simulink model "im_model_exercise_version"  (Simulink 9.2)
settings: Solver=ode45  StartTime=0.0  StopTime=2  MaxStep=300e-6  RelTol=1e-5  EnableMultiTasking=on
InitFcn:
  | Motor_parameters_project
values from neighbouring files (symbols this model uses):
  In = 189    [Motor_parameters_project.m]
  J = 0.0151    [Motor_parameters_project.m]
  Lm = 0.38e-3    (= 0.00038)    [Motor_parameters_project.m]
  Lr = Lm + Ldr    (= 0.00041116)    [Motor_parameters_project.m]
  Ls = Lm + Lds    (= 0.00041116)    [Motor_parameters_project.m]
  Omegae = 2*pi*fn    (= 364.424747816)    [Motor_parameters_project.m]
  p = 2.0    (= 2)    [Motor_parameters_project.m]
  Rr = 2.69e-3    (= 0.00269)    [Motor_parameters_project.m]
  Rs = 2.5e-3    (= 0.0025)    [Motor_parameters_project.m]
  T_rated = Pn/(2*pi*nn/60)    (= 30.0363631473)    [Motor_parameters_project.m]
  Un = 24/sqrt(3)    [Motor_parameters_project.m]
Description:
  | Induction machine model as in Kaz. p 34
  | 
  | Note errors in (1.128) for rotor equations (Lm->Lr for some terms)!
settings Model: Creator=Michael M. Bech  LastModifiedBy=estef  ExtModeTrigMode=oneshot  ExtModeArmWhenConnect=off
settings SolverCC: AlgebraicLoopSolver=LineSearch
settings DataIOCC: LimitDataPoints=off
settings OptimizationCC: BlockReduction=off  BooleanDataType=off  ExpressionDepthLimit=2147483647  InitFltsAndDblsToZero=on
settings DebuggingCC: SaveWithParameterizedLinksMsg=none  SignalResolutionControl=TryResolveAllWithWarning  MultiTaskDSMMsg=warning  MultiTaskCondExecSysMsg=none
settings HardwareCC: TargetUnknown=on
settings GRTTargetCC: TargetFcnLib=ansi_tfl_tmw.mat
settings ConfigComp: CovSFcnEnable=off

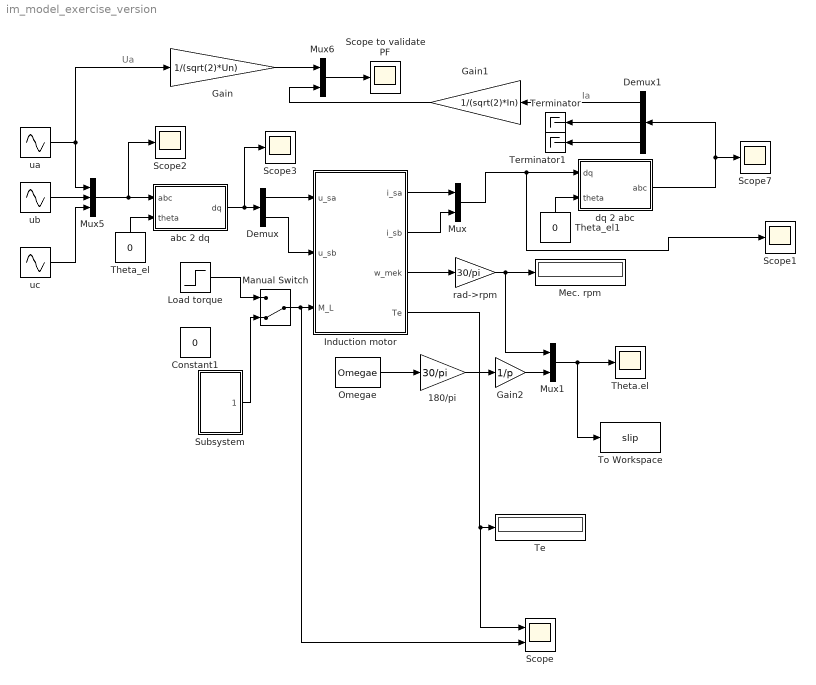
== system im_model_exercise_version ==
  note: Ua
  note: Ia
  180/pi : Gain  Gain=30/pi
  Constant1 : Constant  Value=0
  Demux : Demux  Outputs=2
  Demux1 : Demux  Outputs=3
  Gain : Gain  Gain=1/(sqrt(2)*Un)
  Gain1 : Gain  Gain=1/(sqrt(2)*In)
  Gain2 : Gain  Gain=1/p
  Induction motor : Subsystem
  Load torque : Step  Time=0.25  After=T_rated  SampleTime=0
  Manual Switch : ManualSwitch  CurrentSetting=0
  Mec. rpm : Display
  Mux : Mux  Inputs=2
  Mux1 : Mux  Inputs=2
  Mux5 : Mux  Inputs=3
  Mux6 : Mux  Inputs=2
  Omegae : Constant  Value=Omegae
  Scope : Scope  NumInputPorts=2
  Scope to validate PF : Scope
  Scope{1..3,7} (4 alike) : Scope
  Subsystem : Subsystem
  Te : Display
  Terminator : Terminator
  Terminator1 : Terminator
  Theta.el : Scope
  Theta_el : Constant  Value=0
  Theta_el1 : Constant  Value=0
  To Workspace : ToWorkspace  VariableName=slip  SaveFormat=Timeseries  SampleTime=-1
  abc 2 dq : Subsystem
  dq 2 abc : Subsystem
  rad->rpm : Gain  Gain=30/pi  SaturateOnIntegerOverflow=on  OutDataTypeStr=Inherit: Same as input  ParamDataTypeStr=Inherit: Same as input
  ua : Sin  Amplitude=sqrt(2)*Un  Frequency=Omegae  Phase=pi/2  SampleTime=0
  ub : Sin  Amplitude=sqrt(2)*Un  Frequency=Omegae  Phase=pi/2-120/180*pi  SampleTime=0
  uc : Sin  Amplitude=sqrt(2)*Un  Frequency=Omegae  Phase=pi/2-240/180*pi  SampleTime=0
  wires:
  Induction motor/1(i_sa) -> Mux/1
  Induction motor/2(i_sb) -> Mux/2
  Mux/1 -> dq 2 abc/1(dq), Scope1/1
  Induction motor/3(w_mek) -> rad->rpm/1
  rad->rpm/1 -> Mux1/1, Mec. rpm/1
  abc 2 dq/1(dq) -> Scope3/1, Demux/1
  Demux/2 -> Induction motor/2(u_sb)
  ua/1 -> Mux5/1, Gain/1
  uc/1 -> Mux5/3
  ub/1 -> Mux5/2
  Mux5/1 -> Scope2/1, abc 2 dq/1(abc)
  Theta_el/1 -> abc 2 dq/2(theta)
  Demux/1 -> Induction motor/1(u_sa)
  Theta_el1/1 -> dq 2 abc/2(theta)
  dq 2 abc/1(abc) -> Demux1/1, Scope7/1
  Mux6/1 -> Scope to validate PF/1
  Gain/1 -> Mux6/1
  Demux1/2 -> Terminator/1
  Demux1/3 -> Terminator1/1
  Demux1/1 -> Gain1/1
  Gain1/1 -> Mux6/2
  Load torque/1 -> Manual Switch/1
  Manual Switch/1 -> Scope/2, Induction motor/3(M_L)
  Omegae/1 -> 180/pi/1
  180/pi/1 -> Gain2/1
  Gain2/1 -> Mux1/2
  Mux1/1 -> To Workspace/1, Theta.el/1
  Induction motor/4(Te) -> Scope/1, Te/1
  Subsystem/1(T_load) -> Manual Switch/2

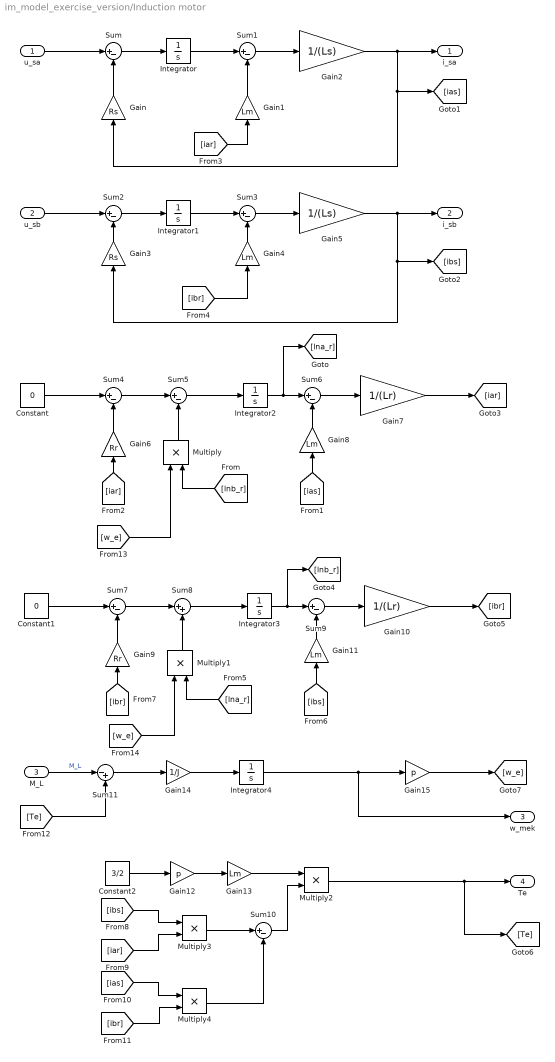
== system im_model_exercise_version/Induction motor ==
  u_sa : Inport
  u_sb : Inport  Port=2
  M_L : Inport  Port=3
  Constant : Constant  Value=0
  Constant1 : Constant  Value=0
  Constant2 : Constant  Value=3/2
  Gain : Gain  Gain=Rs
  Gain{1,4,8,11,13} (5 alike) : Gain  Gain=Lm
  Gain10 : Gain  Gain=1/(Lr)
  Gain12 : Gain  Gain=p
  Gain14 : Gain  Gain=1/J
  Gain15 : Gain  Gain=p
  Gain2 : Gain  Gain=1/(Ls)
  Gain3 : Gain  Gain=Rs
  Gain5 : Gain  Gain=1/(Ls)
  Gain6 : Gain  Gain=Rr
  Gain7 : Gain  Gain=1/(Lr)
  Gain9 : Gain  Gain=Rr
  Integrator{,1..4} (5 alike) : Integrator
  Multiply{,1..4} (5 alike) : Product
  Sum{,1..7,9..10} (10 alike) : Sum  Inputs=|+-
  Sum11 : Sum  Inputs=|-+
  Sum8 : Sum  Inputs=|++
  i_sa : Outport
  i_sb : Outport  Port=2
  w_mek : Outport  Port=3
  Te : Outport  Port=4
  wires:
  u_sa/1 -> Sum/1
  Gain/1 -> Sum/2
  Sum/1 -> Integrator/1
  Integrator/1 -> Sum1/1
  Gain1/1 -> Sum1/2
  Sum1/1 -> Gain2/1
  Gain2/1 -> [ias], Gain/1, i_sa/1
  Gain3/1 -> Sum2/2
  u_sb/1 -> Sum2/1
  Sum3/1 -> Gain5/1
  Gain4/1 -> Sum3/2
  Gain5/1 -> i_sb/1, [ibs], Gain3/1
  Sum2/1 -> Integrator1/1
  Integrator1/1 -> Sum3/1
  Constant/1 -> Sum4/1
  Gain6/1 -> Sum4/2
  Sum4/1 -> Sum5/1
  [lnb_r] -> Multiply/2
  Sum5/1 -> Integrator2/1
  Gain8/1 -> Sum6/2
  [ias] -> Gain8/1
  Integrator2/1 -> [lna_r], Sum6/1
  Sum6/1 -> Gain7/1
  Multiply/1 -> Sum5/2
  Gain7/1 -> [iar]
  [iar] -> Gain6/1
  [ibr] -> Gain4/1
  [iar] -> Gain1/1
  Gain11/1 -> Sum9/2
  Gain10/1 -> [ibr]
  [ibr] -> Gain9/1
  [ibs] -> Gain11/1
  Multiply1/1 -> Sum8/2
  Integrator3/1 -> [lnb_r], Sum9/1
  Sum7/1 -> Sum8/1
  [lna_r] -> Multiply1/2
  Gain9/1 -> Sum7/2
  Sum9/1 -> Gain10/1
  Sum8/1 -> Integrator3/1
  Constant1/1 -> Sum7/1
  Gain13/1 -> Multiply2/1
  Sum10/1 -> Multiply2/2
  [ibs] -> Multiply3/1
  [iar] -> Multiply3/2
  Multiply3/1 -> Sum10/1
  [ias] -> Multiply4/1
  [ibr] -> Multiply4/2
  Multiply4/1 -> Sum10/2
  Constant2/1 -> Gain12/1
  Gain12/1 -> Gain13/1
  Multiply2/1 -> [Te], Te/1
  [Te] -> Sum11/2
  M_L/1 -> Sum11/1  "M_L"
  Sum11/1 -> Gain14/1
  Gain14/1 -> Integrator4/1
  Integrator4/1 -> Gain15/1, w_mek/1
  Gain15/1 -> [w_e]
  [w_e] -> Multiply1/1
  [w_e] -> Multiply/1

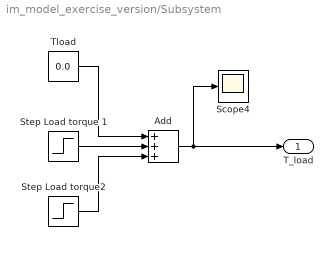
== system im_model_exercise_version/Subsystem ==
  Add : Sum  Inputs=+++
  Scope4 : Scope
  Step Load torque 1 : Step  Time=0.9  After=5  SampleTime=0
  Step Load torque2 : Step  Time=1.8  After=25  SampleTime=0
  Tload : Constant  Value=0.0
  T_load : Outport
  wires:
  Add/1 -> T_load/1, Scope4/1
  Step Load torque 1/1 -> Add/2
  Tload/1 -> Add/1
  Step Load torque2/1 -> Add/3

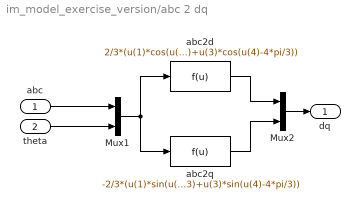
== system im_model_exercise_version/abc 2 dq ==
  abc : Inport
  theta : Inport  Port=2
  Mux1 : Mux  Inputs=2
  Mux2 : Mux  Inputs=2
  abc2d : Fcn  Expr=2/3*(u(1)*cos(u(4))+u(2)*cos(u(4)-2*pi/3)+u(3)*cos(u(4)-4*pi/3))
  abc2q : Fcn  Expr=-2/3*(u(1)*sin(u(4))+u(2)*sin(u(4)-2*pi/3)+u(3)*sin(u(4)-4*pi/3))
  dq : Outport
  wires:
  abc/1 -> Mux1/1
  theta/1 -> Mux1/2
  Mux1/1 -> abc2d/1, abc2q/1
  abc2d/1 -> Mux2/1
  abc2q/1 -> Mux2/2
  Mux2/1 -> dq/1

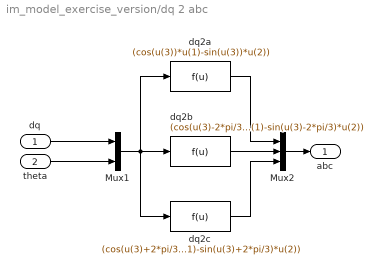
== system im_model_exercise_version/dq 2 abc ==
  dq : Inport
  theta : Inport  Port=2
  Mux1 : Mux  Inputs=2
  Mux2 : Mux  Inputs=3
  dq2a : Fcn  Expr=(cos(u(3))*u(1)-sin(u(3))*u(2))
  dq2b : Fcn  Expr=(cos(u(3)-2*pi/3)*u(1)-sin(u(3)-2*pi/3)*u(2))
  dq2c : Fcn  Expr=(cos(u(3)+2*pi/3)*u(1)-sin(u(3)+2*pi/3)*u(2))
  abc : Outport
  wires:
  Mux2/1 -> abc/1
  dq2b/1 -> Mux2/2
  dq2a/1 -> Mux2/1
  Mux1/1 -> dq2a/1, dq2c/1, dq2b/1
  theta/1 -> Mux1/2
  dq/1 -> Mux1/1
  dq2c/1 -> Mux2/3
